simulink model "QuadrotorSimulink_no_memory"  (R2020a)
settings: Solver=FixedStepAuto  StartTime=0.0  StopTime=options.T_train  FixedStep=options.dt  RelTol=1e-6
undefined symbols (not defined in the file or in its folder): options, Quad
libraries: neural x67, simulink x1
(part 1 of 4)
settings Model: Creator=test  LastModifiedBy=kekatos
settings DataIOCC: LimitDataPoints=on  SaveFormat=Array  SignalLoggingSaveFormat=ModelDataLogs  ReturnWorkspaceOutputs=off
settings OptimizationCC: ExpressionDepthLimit=2147483647  LifeSpan=inf
settings DebuggingCC: UnderspecifiedInitializationDetection=Classic  MergeDetectMultiDrivingBlocksExec=none  SolverPrmCheckMsg=warning  FcnCallInpInsideContextMsg=warning  StateNameClashWarn=warning  SFUnexpectedBacktrackingDiag=warning  SFNoUnconditionalDefaultTransitionDiag=warning  SFExecutionAtInitializationDiag=none  ArithmeticOperatorsInVariantConditions=warning
settings HardwareCC: ProdBitPerPointer=32  ProdBitPerSizeT=32  ProdBitPerPtrDiffT=32  ProdLargestAtomicFloat=None  ProdIntDivRoundTo=Undefined  ProdEndianess=Unspecified  ProdWordSize=32  ProdHWDeviceType=32-bit Generic
settings ModelReferenceCC: PropagateSignalLabelsOutOfModel=off
settings SFSimCC: SimUseLocalCustomCode=off  CustomCodeUndefinedFunction=UseInterfaceOnly
settings RTWCC: RTWUseLocalCustomCode=off
settings CodeAppCC: StateflowObjectComments=on
settings GRTTargetCC: TargetLangStandard=C89/C90 (ANSI)  CombineOutputUpdateFcns=off  GRTInterface=on
settings ConfigComp: CovMetricSettings=dw  CovHtmlReporting=on  CovSaveCumulativeToWorkspaceVar=on  CovSaveSingleToWorkspaceVar=on

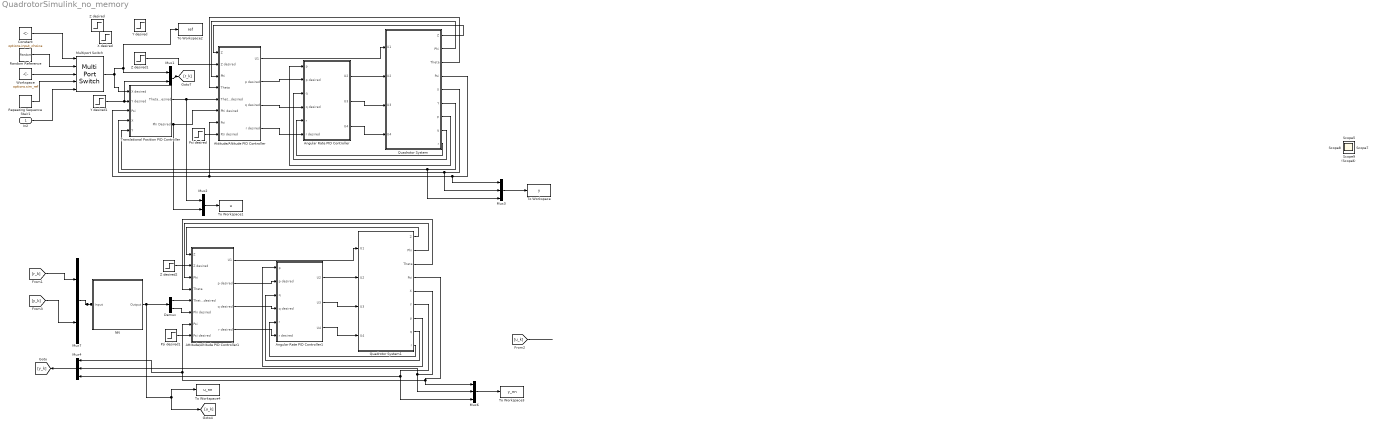
== system QuadrotorSimulink_no_memory ==
  In2 : Inport
  Angular Rate PID Controller : Subsystem
  Angular Rate PID Controller1 : Subsystem
  Attitude/Altitude PID Controller : Subsystem
  Attitude/Altitude PID Controller1 : Subsystem
  Constant : Constant  Value=options.input_choice
  Demux : Demux  Outputs=2
  Multiport Switch : MultiPortSwitch  Inputs=4
  Mux1 : Mux  Inputs=2
  Mux2 : Mux  Inputs=2
  Mux3 : Mux  Inputs=3
  Mux4 : Mux  Inputs=3
  Mux6 : Mux  Inputs=3
  Mux7 : Mux  Inputs=2
  NN : Subsystem
      mask help: Feed-Forward Neural Network
      mask Display: e = 0.06;c1 = [120 150 230]/255;c2 = ([120 150 230]+0)/383;c3 = ([120 150 230]+128)/383;patch([0 1 1 0],[0 0 1 1],c1);patch([0 1 1 1-e 1-e 0+e],[0 0 1 1-e 0+e 0+e],c2);patch([0 0 1 1-e 0+e 0+e],[0 1 1 1-e 1-e 0+e],c3);plot([0 1 1 0 0],[0 0 1 1 0]);fprintf('NNET');port_label('input',1,' Input');port_label('output',1,'Output ');
  Psi desired : Step  After=0  SampleTime=0
  Psi desired1 : Step  After=0  SampleTime=0
  Quadrotor System : Subsystem
  Quadrotor System1 : Subsystem
  Random Reference : UniformRandomNumber  Minimum=options.ref_min  Maximum=options.ref_max  Seed=randi(2^32,[1 ])  SampleTime=options.ref_Ts
  Repeating Sequence Stair1 : simulink/Sources/Repeating Sequence Stair  OutValues=options.sim_cov  tsamp=options.ref_Ts  OutMin=[]  OutMax=[]  OutDataTypeStr=double  OutputDataTypeScalingMode=double  OutDataType=fixdt(0,8)  ConRadixGroup=Best Precision: Vector-wise  OutScaling=2^-12
  To Workspace : ToWorkspace  VariableName=y  SaveFormat=Structure With Time  SampleTime=0.01
  To Workspace1 : ToWorkspace  VariableName=u  SaveFormat=Structure With Time  SampleTime=0.01
  To Workspace2 : ToWorkspace  VariableName=ref  SaveFormat=Structure With Time  SampleTime=0.01
  To Workspace3 : ToWorkspace  VariableName=y_nn  SaveFormat=Structure With Time  SampleTime=0.01
  To Workspace4 : ToWorkspace  VariableName=u_nn  SaveFormat=Structure With Time  SampleTime=0.01
  Translational Position PID Controller : Subsystem
  Workspace : Constant  Value=options.sim_ref
  X desired : Step  After=.25  SampleTime=0
  Y desired : Step  After=0  SampleTime=0
  Y desired1 : Step  Time=0  After=0.05  SampleTime=0
  Z desired : Step  After=.5  SampleTime=0
  Z desired1 : Step  Time=0  After=0.5  SampleTime=0
  Z desired2 : Step  Time=0  After=0.5  SampleTime=0
  Scope{,1..10} (11 alike) : Scope
  wires:
  Quadrotor System/2(Phi) -> Attitude/Altitude PID Controller/3(Phi)
  Quadrotor System/3(Theta) -> Attitude/Altitude PID Controller/4(Theta)
  Quadrotor System/4(Psi) -> Mux3/1, Translational Position PID Controller/3(Psi), Attitude/Altitude PID Controller/7(Psi)
  Quadrotor System/5(X) -> Mux3/2, Translational Position PID Controller/4(X)
  Quadrotor System/6(Y) -> Mux3/3, Translational Position PID Controller/5(Y)
  Quadrotor System/1(Z) -> Attitude/Altitude PID Controller/1(Z)
  Psi desired/1 -> Attitude/Altitude PID Controller/8(Psi desired)
  Attitude/Altitude PID Controller/1(U1) -> Quadrotor System/1(U1)
  Translational Position PID Controller/1(Theta Desired) -> Mux2/1, Attitude/Altitude PID Controller/5(Theta desired)
  Translational Position PID Controller/2(Phi Desired) -> Attitude/Altitude PID Controller/6(Phi desired), Mux2/2
  Attitude/Altitude PID Controller/2(p desired) -> Angular Rate PID Controller/2(p desired)
  Attitude/Altitude PID Controller/3(q desired) -> Angular Rate PID Controller/4(q desired)
  Attitude/Altitude PID Controller/4(r desired) -> Angular Rate PID Controller/6(r desired)
  Quadrotor System/9(r) -> Angular Rate PID Controller/5(r)
  Quadrotor System/8(q) -> Angular Rate PID Controller/3(q)
  Quadrotor System/7(p) -> Angular Rate PID Controller/1(p)
  Angular Rate PID Controller/3(U4) -> Quadrotor System/4(U4)
  Angular Rate PID Controller/2(U3) -> Quadrotor System/3(U3)
  Angular Rate PID Controller/1(U2) -> Quadrotor System/2(U2)
  Y desired1/1 -> Mux1/2, Translational Position PID Controller/2(Y desired)
  Z desired1/1 -> Attitude/Altitude PID Controller/2(Z desired)
  Mux2/1 -> To Workspace1/1
  Mux3/1 -> To Workspace/1
  In2/1 -> Multiport Switch/5
  Workspace/1 -> Multiport Switch/3
  Random Reference/1 -> Multiport Switch/2
  Repeating Sequence Stair1/1 -> Multiport Switch/4
  Constant/1 -> Multiport Switch/1
  Attitude/Altitude PID Controller1/2(p desired) -> Angular Rate PID Controller1/2(p desired)
  Attitude/Altitude PID Controller1/1(U1) -> Quadrotor System1/1(U1)
  Psi desired1/1 -> Attitude/Altitude PID Controller1/8(Psi desired)
  Quadrotor System1/9(r) -> Angular Rate PID Controller1/5(r)
  Quadrotor System1/6(Y) -> Mux4/3, Mux6/3
  Angular Rate PID Controller1/2(U3) -> Quadrotor System1/3(U3)
  Demux/1 -> Attitude/Altitude PID Controller1/5(Theta desired)
  Attitude/Altitude PID Controller1/3(q desired) -> Angular Rate PID Controller1/4(q desired)
  Quadrotor System1/7(p) -> Angular Rate PID Controller1/1(p)
  Quadrotor System1/2(Phi) -> Attitude/Altitude PID Controller1/3(Phi)
  Z desired2/1 -> Attitude/Altitude PID Controller1/2(Z desired)
  Quadrotor System1/4(Psi) -> Mux6/1, Mux4/1, Attitude/Altitude PID Controller1/7(Psi)
  Demux/2 -> Attitude/Altitude PID Controller1/6(Phi desired)
  Quadrotor System1/3(Theta) -> Attitude/Altitude PID Controller1/4(Theta)
  Angular Rate PID Controller1/1(U2) -> Quadrotor System1/2(U2)
  Quadrotor System1/5(X) -> Mux4/2, Mux6/2
  Angular Rate PID Controller1/3(U4) -> Quadrotor System1/4(U4)
  Quadrotor System1/1(Z) -> Attitude/Altitude PID Controller1/1(Z)
  Attitude/Altitude PID Controller1/4(r desired) -> Angular Rate PID Controller1/6(r desired)
  NN/1(Output) -> [u_k], To Workspace4/1, Demux/1
  Mux6/1 -> To Workspace3/1
  Quadrotor System1/8(q) -> Angular Rate PID Controller1/3(q)
  Mux7/1 -> NN/1(Input)
  Multiport Switch/1 -> Translational Position PID Controller/1(X desired), To Workspace2/1, Mux1/1
  Mux4/1 -> [y_k]
  [r_k] -> Mux7/1
  [u_k] -> ?
  Mux1/1 -> [r_k]
  [y_k] -> Mux7/2

== system QuadrotorSimulink_no_memory/Angular Rate PID Controller ==
  p : Inport
  p desired : Inport  Port=2
  q : Inport  Port=3
  q desired : Inport  Port=4
  r : Inport  Port=5
  r desired : Inport  Port=6
  p PID : Subsystem
  q PID : Subsystem
  r PID : Subsystem
  U2 : Outport  VectorParamsAs1DForOutWhenUnconnected=off
  U3 : Outport  Port=2  VectorParamsAs1DForOutWhenUnconnected=off
  U4 : Outport  Port=3  VectorParamsAs1DForOutWhenUnconnected=off
  wires:
  p PID/1(U2) -> U2/1
  q PID/1(U3) -> U3/1
  r PID/1(U4) -> U4/1
  p/1 -> p PID/1(p)
  p desired/1 -> p PID/2(p desired)
  q/1 -> q PID/1(q)
  q desired/1 -> q PID/2(q desired)
  r/1 -> r PID/1(r)
  r desired/1 -> r PID/2(r desired)

== system QuadrotorSimulink_no_memory/Angular Rate PID Controller1 ==
  p : Inport
  p desired : Inport  Port=2
  q : Inport  Port=3
  q desired : Inport  Port=4
  r : Inport  Port=5
  r desired : Inport  Port=6
  p PID : Subsystem
  q PID : Subsystem
  r PID : Subsystem
  U2 : Outport  VectorParamsAs1DForOutWhenUnconnected=off
  U3 : Outport  Port=2  VectorParamsAs1DForOutWhenUnconnected=off
  U4 : Outport  Port=3  VectorParamsAs1DForOutWhenUnconnected=off
  wires:
  p PID/1(U2) -> U2/1
  q PID/1(U3) -> U3/1
  r PID/1(U4) -> U4/1
  p/1 -> p PID/1(p)
  p desired/1 -> p PID/2(p desired)
  q/1 -> q PID/1(q)
  q desired/1 -> q PID/2(q desired)
  r/1 -> r PID/1(r)
  r desired/1 -> r PID/2(r desired)

== system QuadrotorSimulink_no_memory/Attitude//Altitude PID Controller ==
  Z : Inport
  Z desired : Inport  Port=2
  Phi : Inport  Port=3
  Theta : Inport  Port=4
  Theta desired : Inport  Port=5
  Phi desired : Inport  Port=6
  Psi : Inport  Port=7
  Psi desired : Inport  Port=8
  Phi PID : Subsystem
  Psi PID : Subsystem
  Theta PID : Subsystem
  Z PID : Subsystem
  U1 : Outport  VectorParamsAs1DForOutWhenUnconnected=off
  p desired : Outport  Port=2  VectorParamsAs1DForOutWhenUnconnected=off
  q desired : Outport  Port=3  VectorParamsAs1DForOutWhenUnconnected=off
  r desired : Outport  Port=4  VectorParamsAs1DForOutWhenUnconnected=off
  wires:
  Z PID/1(U1) -> U1/1
  Z desired/1 -> Z PID/2(Z desired)
  Z/1 -> Z PID/1(Z)
  Phi desired/1 -> Phi PID/2(Phi desired)
  Phi/1 -> Phi PID/1(Phi), Z PID/3(Phi)
  Psi desired/1 -> Psi PID/2(Psi desired)
  Psi/1 -> Psi PID/1(Psi)
  Theta desired/1 -> Theta PID/2(Theta desired)
  Theta/1 -> Theta PID/1(Theta), Z PID/4(Theta)
  Phi PID/1(p desired) -> p desired/1
  Psi PID/1(r desired) -> r desired/1
  Theta PID/1(q desired) -> q desired/1

== system QuadrotorSimulink_no_memory/Attitude//Altitude PID Controller1 ==
  Z : Inport
  Z desired : Inport  Port=2
  Phi : Inport  Port=3
  Theta : Inport  Port=4
  Theta desired : Inport  Port=5
  Phi desired : Inport  Port=6
  Psi : Inport  Port=7
  Psi desired : Inport  Port=8
  Phi PID : Subsystem
  Psi PID : Subsystem
  Theta PID : Subsystem
  Z PID : Subsystem
  U1 : Outport  VectorParamsAs1DForOutWhenUnconnected=off
  p desired : Outport  Port=2  VectorParamsAs1DForOutWhenUnconnected=off
  q desired : Outport  Port=3  VectorParamsAs1DForOutWhenUnconnected=off
  r desired : Outport  Port=4  VectorParamsAs1DForOutWhenUnconnected=off
  wires:
  Z PID/1(U1) -> U1/1
  Z desired/1 -> Z PID/2(Z desired)
  Z/1 -> Z PID/1(Z)
  Phi desired/1 -> Phi PID/2(Phi desired)
  Phi/1 -> Phi PID/1(Phi), Z PID/3(Phi)
  Psi desired/1 -> Psi PID/2(Psi desired)
  Psi/1 -> Psi PID/1(Psi)
  Theta desired/1 -> Theta PID/2(Theta desired)
  Theta/1 -> Theta PID/1(Theta), Z PID/4(Theta)
  Phi PID/1(p desired) -> p desired/1
  Psi PID/1(r desired) -> r desired/1
  Theta PID/1(q desired) -> q desired/1

== system QuadrotorSimulink_no_memory/NN ==
  Input : Inport  PortDimensions=5
      mask Display: e = 0.06;c1 = [120 230 180]/255;c2 = ([120 230 180]+0)/(256+128);c3 = ([120 230 180]+128)/(256+128);patch([0 1 1 0],[0 0 1 1],c1);patch([0 1 1 1-e 1-e 0+e],[0 0 1 1-e 0+e 0+e],c2);patch([0 0 1 1-e 0+e 0+e],[0 1 1 1-e 1-e 0+e],c3);plot([0 1 1 0 0],[0 0 1 1 0]);
  Layer 1 : Subsystem
      mask Display: e = 0.06;c1 = [120 150 230]/255;c2 = ([120 150 230]+0)/383;c3 = ([120 150 230]+128)/383;patch([0 1 1 0],[0 0 1 1],c1);patch([0 1 1 1-e 1-e 0+e],[0 0 1 1-e 0+e 0+e],c2);patch([0 0 1 1-e 0+e 0+e],[0 1 1 1-e 1-e 0+e],c3);plot([0 1 1 0 0],[0 0 1 1 0]);
  Layer 2 : Subsystem
      mask Display: e = 0.06;c1 = [120 150 230]/255;c2 = ([120 150 230]+0)/383;c3 = ([120 150 230]+128)/383;patch([0 1 1 0],[0 0 1 1],c1);patch([0 1 1 1-e 1-e 0+e],[0 0 1 1-e 0+e 0+e],c2);patch([0 0 1 1-e 0+e 0+e],[0 1 1 1-e 1-e 0+e],c3);plot([0 1 1 0 0],[0 0 1 1 0]);
  Layer 3 : Subsystem
      mask Display: e = 0.06;c1 = [120 150 230]/255;c2 = ([120 150 230]+0)/383;c3 = ([120 150 230]+128)/383;patch([0 1 1 0],[0 0 1 1],c1);patch([0 1 1 1-e 1-e 0+e],[0 0 1 1-e 0+e 0+e],c2);patch([0 0 1 1-e 0+e 0+e],[0 1 1 1-e 1-e 0+e],c3);plot([0 1 1 0 0],[0 0 1 1 0]);
  Process Input 1 : Subsystem
      mask Display: e = 0.06;c1 = [120 150 230]/255;c2 = ([120 150 230]+0)/383;c3 = ([120 150 230]+128)/383;patch([0 1 1 0],[0 0 1 1],c1);patch([0 1 1 1-e 1-e 0+e],[0 0 1 1-e 0+e 0+e],c2);patch([0 0 1 1-e 0+e 0+e],[0 1 1 1-e 1-e 0+e],c3);plot([0 1 1 0 0],[0 0 1 1 0]);
  Process Output 1 : Subsystem
      mask Display: e = 0.06;c1 = [120 150 230]/255;c2 = ([120 150 230]+0)/383;c3 = ([120 150 230]+128)/383;patch([0 1 1 0],[0 0 1 1],c1);patch([0 1 1 1-e 1-e 0+e],[0 0 1 1-e 0+e 0+e],c2);patch([0 0 1 1-e 0+e 0+e],[0 1 1 1-e 1-e 0+e],c3);plot([0 1 1 0 0],[0 0 1 1 0]);
  Output : Outport  InitialOutput=[0;0]
      mask Display: e = 0.06;c1 = [120 230 180]/255;c2 = ([120 230 180]+0)/(256+128);c3 = ([120 230 180]+128)/(256+128);patch([0 1 1 0],[0 0 1 1],c1);patch([0 1 1 1-e 1-e 0+e],[0 0 1 1-e 0+e 0+e],c2);patch([0 0 1 1-e 0+e 0+e],[0 1 1 1-e 1-e 0+e],c3);plot([0 1 1 0 0],[0 0 1 1 0]);
  wires:
  Input/1 -> Process Input 1/1(x)
  Process Output 1/1(y) -> Output/1
  Process Input 1/1(p) -> Layer 1/1("p{1}")
  Layer 1/1("a{1}") -> [feedback1]
  [feedback1] -> Layer 2/1("a{1} ")
  Layer 2/1("a{2}") -> [feedback2]
  [feedback2] -> Layer 3/1("a{2} ")
  Layer 3/1("a{3}") -> Process Output 1/1(a)

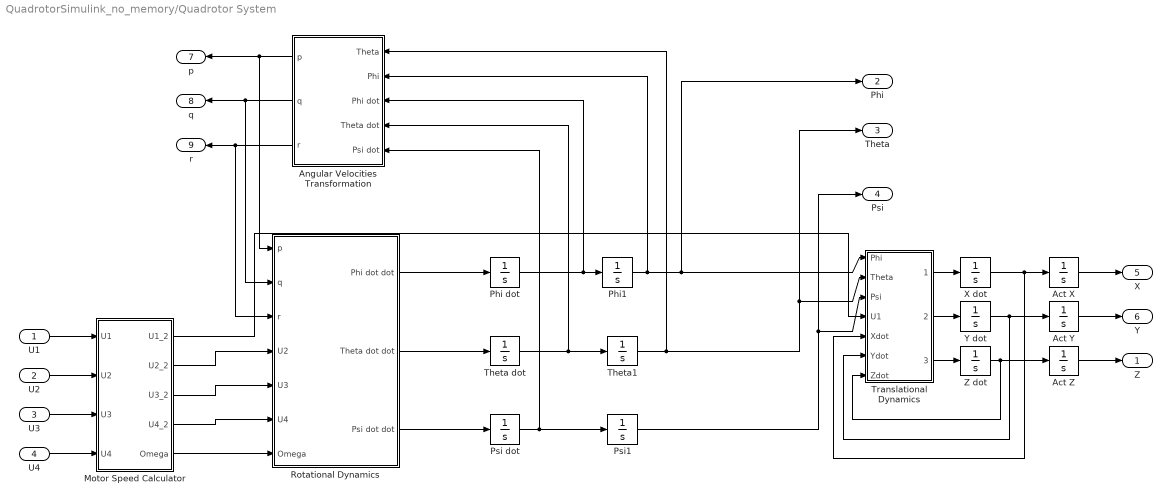
== system QuadrotorSimulink_no_memory/Quadrotor System ==
  U1 : Inport
  U2 : Inport  Port=2
  U3 : Inport  Port=3
  U4 : Inport  Port=4
  Act X : Integrator
  Act Y : Integrator
  Act Z : Integrator
  Angular Velocities Transformation : Subsystem
  Motor Speed Calculator : Subsystem
  Phi dot : Integrator
  Phi1 : Integrator  ZeroCross=off
  Psi dot : Integrator  ZeroCross=off
  Psi1 : Integrator  ZeroCross=off
  Rotational Dynamics : Subsystem
  Theta dot : Integrator  ZeroCross=off
  Theta1 : Integrator  ZeroCross=off
  Translational Dynamics : Subsystem
  X dot : Integrator
  Y dot : Integrator
  Z dot : Integrator
  Z : Outport  VectorParamsAs1DForOutWhenUnconnected=off
  Phi : Outport  Port=2  VectorParamsAs1DForOutWhenUnconnected=off
  Theta : Outport  Port=3  VectorParamsAs1DForOutWhenUnconnected=off
  Psi : Outport  Port=4  VectorParamsAs1DForOutWhenUnconnected=off
  X : Outport  Port=5  VectorParamsAs1DForOutWhenUnconnected=off
  Y : Outport  Port=6  VectorParamsAs1DForOutWhenUnconnected=off
  p : Outport  Port=7  VectorParamsAs1DForOutWhenUnconnected=off
  q : Outport  Port=8  VectorParamsAs1DForOutWhenUnconnected=off
  r : Outport  Port=9  VectorParamsAs1DForOutWhenUnconnected=off
  wires:
  Rotational Dynamics/2(Theta dot dot) -> Theta dot/1
  Motor Speed Calculator/5(Omega) -> Rotational Dynamics/7(Omega)
  Phi1/1 -> Translational Dynamics/1(Phi), Phi/1, Angular Velocities Transformation/2(Phi)
  Theta1/1 -> Translational Dynamics/2(Theta), Theta/1, Angular Velocities Transformation/1(Theta)
  Psi1/1 -> Translational Dynamics/3(Psi), Psi/1
  Translational Dynamics/1(x dotdot) -> X dot/1
  X dot/1 -> Act X/1, Translational Dynamics/5(Xdot)
  Y dot/1 -> Act Y/1, Translational Dynamics/6(Ydot)
  Translational Dynamics/2(y dotdot) -> Y dot/1
  Z dot/1 -> Translational Dynamics/7(Zdot), Act Z/1
  Translational Dynamics/3(z dotdot) -> Z dot/1
  Act X/1 -> X/1
  Act Y/1 -> Y/1
  Act Z/1 -> Z/1
  Psi dot/1 -> Psi1/1, Angular Velocities Transformation/5(Psi dot)
  Theta dot/1 -> Theta1/1, Angular Velocities Transformation/4(Theta dot)
  Phi dot/1 -> Phi1/1, Angular Velocities Transformation/3(Phi dot)
  Rotational Dynamics/3(Psi dot dot) -> Psi dot/1
  Rotational Dynamics/1(Phi dot dot) -> Phi dot/1
  U4/1 -> Motor Speed Calculator/4(U4)
  U2/1 -> Motor Speed Calculator/2(U2)
  U3/1 -> Motor Speed Calculator/3(U3)
  Motor Speed Calculator/2(U2_2) -> Rotational Dynamics/4(U2)
  Motor Speed Calculator/3(U3_2) -> Rotational Dynamics/5(U3)
  Motor Speed Calculator/1(U1_2) -> Translational Dynamics/4(U1)
  Motor Speed Calculator/4(U4_2) -> Rotational Dynamics/6(U4)
  Angular Velocities Transformation/1(p) -> Rotational Dynamics/1(p), p/1
  Angular Velocities Transformation/2(q) -> Rotational Dynamics/2(q), q/1
  Angular Velocities Transformation/3(r) -> Rotational Dynamics/3(r), r/1
  U1/1 -> Motor Speed Calculator/1(U1)

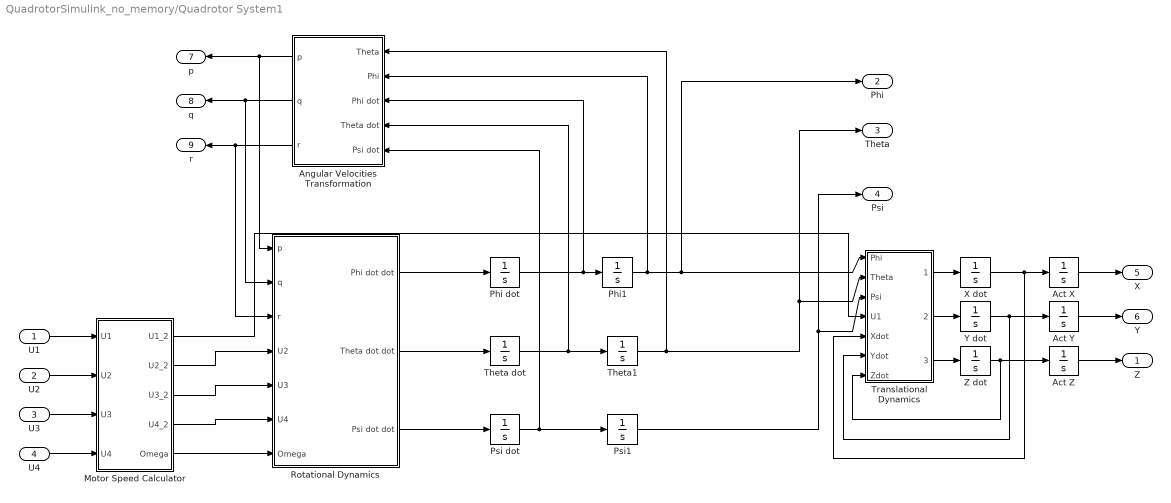
== system QuadrotorSimulink_no_memory/Quadrotor System1 ==
  U1 : Inport
  U2 : Inport  Port=2
  U3 : Inport  Port=3
  U4 : Inport  Port=4
  Act X : Integrator
  Act Y : Integrator
  Act Z : Integrator
  Angular Velocities Transformation : Subsystem
  Motor Speed Calculator : Subsystem
  Phi dot : Integrator
  Phi1 : Integrator  ZeroCross=off
  Psi dot : Integrator  ZeroCross=off
  Psi1 : Integrator  ZeroCross=off
  Rotational Dynamics : Subsystem
  Theta dot : Integrator  ZeroCross=off
  Theta1 : Integrator  ZeroCross=off
  Translational Dynamics : Subsystem
  X dot : Integrator
  Y dot : Integrator
  Z dot : Integrator
  Z : Outport  VectorParamsAs1DForOutWhenUnconnected=off
  Phi : Outport  Port=2  VectorParamsAs1DForOutWhenUnconnected=off
  Theta : Outport  Port=3  VectorParamsAs1DForOutWhenUnconnected=off
  Psi : Outport  Port=4  VectorParamsAs1DForOutWhenUnconnected=off
  X : Outport  Port=5  VectorParamsAs1DForOutWhenUnconnected=off
  Y : Outport  Port=6  VectorParamsAs1DForOutWhenUnconnected=off
  p : Outport  Port=7  VectorParamsAs1DForOutWhenUnconnected=off
  q : Outport  Port=8  VectorParamsAs1DForOutWhenUnconnected=off
  r : Outport  Port=9  VectorParamsAs1DForOutWhenUnconnected=off
  wires:
  Rotational Dynamics/2(Theta dot dot) -> Theta dot/1
  Motor Speed Calculator/5(Omega) -> Rotational Dynamics/7(Omega)
  Phi1/1 -> Translational Dynamics/1(Phi), Phi/1, Angular Velocities Transformation/2(Phi)
  Theta1/1 -> Translational Dynamics/2(Theta), Theta/1, Angular Velocities Transformation/1(Theta)
  Psi1/1 -> Translational Dynamics/3(Psi), Psi/1
  Translational Dynamics/1(x dotdot) -> X dot/1
  X dot/1 -> Act X/1, Translational Dynamics/5(Xdot)
  Y dot/1 -> Act Y/1, Translational Dynamics/6(Ydot)
  Translational Dynamics/2(y dotdot) -> Y dot/1
  Z dot/1 -> Translational Dynamics/7(Zdot), Act Z/1
  Translational Dynamics/3(z dotdot) -> Z dot/1
  Act X/1 -> X/1
  Act Y/1 -> Y/1
  Act Z/1 -> Z/1
  Psi dot/1 -> Psi1/1, Angular Velocities Transformation/5(Psi dot)
  Theta dot/1 -> Theta1/1, Angular Velocities Transformation/4(Theta dot)
  Phi dot/1 -> Phi1/1, Angular Velocities Transformation/3(Phi dot)
  Rotational Dynamics/3(Psi dot dot) -> Psi dot/1
  Rotational Dynamics/1(Phi dot dot) -> Phi dot/1
  U4/1 -> Motor Speed Calculator/4(U4)
  U2/1 -> Motor Speed Calculator/2(U2)
  U3/1 -> Motor Speed Calculator/3(U3)
  Motor Speed Calculator/2(U2_2) -> Rotational Dynamics/4(U2)
  Motor Speed Calculator/3(U3_2) -> Rotational Dynamics/5(U3)
  Motor Speed Calculator/1(U1_2) -> Translational Dynamics/4(U1)
  Motor Speed Calculator/4(U4_2) -> Rotational Dynamics/6(U4)
  Angular Velocities Transformation/1(p) -> Rotational Dynamics/1(p), p/1
  Angular Velocities Transformation/2(q) -> Rotational Dynamics/2(q), q/1
  Angular Velocities Transformation/3(r) -> Rotational Dynamics/3(r), r/1
  U1/1 -> Motor Speed Calculator/1(U1)

== system QuadrotorSimulink_no_memory/Translational Position PID Controller ==
  X desired : Inport
  Y desired : Inport  Port=2
  Psi : Inport  Port=3
  X : Inport  Port=4
  Y : Inport  Port=5
  Desired Position GF to BF : Subsystem
  Position GF to BF : Subsystem
  X PID : Subsystem
  Y PID : Subsystem
  Theta Desired : Outport  VectorParamsAs1DForOutWhenUnconnected=off
  Phi Desired : Outport  Port=2  VectorParamsAs1DForOutWhenUnconnected=off
  wires:
  X PID/1(Theta Desired) -> Theta Desired/1
  Y PID/1(Phi Desired) -> Phi Desired/1
  X desired/1 -> Desired Position GF to BF/1(X GF)
  Y desired/1 -> Desired Position GF to BF/2(Y GF)
  Desired Position GF to BF/1("X Bf ") -> X PID/1(X desired)
  Desired Position GF to BF/2(Y Bf) -> Y PID/1(Y desired)
  X/1 -> Position GF to BF/1(X GF)
  Y/1 -> Position GF to BF/2(Y GF)
  Position GF to BF/1("X Bf ") -> X PID/2(X)
  Position GF to BF/2(Y Bf) -> Y PID/2(Y)
  Psi/1 -> Desired Position GF to BF/3(Psi), Position GF to BF/3(Psi)

== system QuadrotorSimulink_no_memory/Angular Rate PID Controller/p PID ==
  p : Inport
  p desired : Inport  Port=2
  Derivative : Derivative
  Integrator : Integrator
  Kd : Gain  Gain=Quad.p_KD
  Ki : Gain  Gain=Quad.p_KI
  Kp : Gain  Gain=Quad.p_KP
  Psi Error : Sum  Inputs=+-
  Saturation1 : Saturate  UpperLimit=Quad.U2_max  LowerLimit=Quad.U2_min
  Sum : Sum  Inputs=+++
  U2 : Outport  VectorParamsAs1DForOutWhenUnconnected=off
  wires:
  p/1 -> Psi Error/2, Derivative/1
  p desired/1 -> Psi Error/1
  Derivative/1 -> Kd/1
  Kp/1 -> Sum/1
  Sum/1 -> U2/1
  Psi Error/1 -> Integrator/1, Kp/1
  Integrator/1 -> Ki/1
  Kd/1 -> Sum/3
  Ki/1 -> Saturation1/1
  Saturation1/1 -> Sum/2

== system QuadrotorSimulink_no_memory/Angular Rate PID Controller/q PID ==
  q : Inport
  q desired : Inport  Port=2
  Derivative : Derivative
  Integrator : Integrator
  Kd : Gain  Gain=Quad.q_KD
  Ki : Gain  Gain=Quad.q_KI
  Kp : Gain  Gain=Quad.q_KP
  Saturation1 : Saturate  UpperLimit=Quad.U3_max  LowerLimit=Quad.U3_min
  Scope : Scope
  Sum : Sum  Inputs=+++
  q Error : Sum  Inputs=+-
  U3 : Outport  VectorParamsAs1DForOutWhenUnconnected=off
  wires:
  q/1 -> q Error/2, Derivative/1
  q desired/1 -> q Error/1
  Derivative/1 -> Kd/1
  Kp/1 -> Sum/1
  Sum/1 -> U3/1
  q Error/1 -> Integrator/1, Kp/1, Scope/1
  Integrator/1 -> Ki/1
  Kd/1 -> Sum/3
  Ki/1 -> Saturation1/1
  Saturation1/1 -> Sum/2

== system QuadrotorSimulink_no_memory/Angular Rate PID Controller/r PID ==
  r : Inport
  r desired : Inport  Port=2
  Derivative : Derivative
  Integrator : Integrator
  Kd : Gain  Gain=Quad.r_KD
  Ki : Gain  Gain=Quad.r_KI
  Kp : Gain  Gain=Quad.r_KP
  Psi Error : Sum  Inputs=+-
  Sum : Sum  Inputs=+++
  U4 : Outport  VectorParamsAs1DForOutWhenUnconnected=off
  wires:
  r/1 -> Psi Error/2, Derivative/1
  r desired/1 -> Psi Error/1
  Derivative/1 -> Kd/1
  Kp/1 -> Sum/1
  Sum/1 -> U4/1
  Psi Error/1 -> Integrator/1, Kp/1
  Integrator/1 -> Ki/1
  Kd/1 -> Sum/3

== system QuadrotorSimulink_no_memory/Angular Rate PID Controller1/p PID ==
  p : Inport
  p desired : Inport  Port=2
  Derivative : Derivative
  Integrator : Integrator
  Kd : Gain  Gain=Quad.p_KD
  Ki : Gain  Gain=Quad.p_KI
  Kp : Gain  Gain=Quad.p_KP
  Psi Error : Sum  Inputs=+-
  Saturation1 : Saturate  UpperLimit=Quad.U2_max  LowerLimit=Quad.U2_min
  Sum : Sum  Inputs=+++
  U2 : Outport  VectorParamsAs1DForOutWhenUnconnected=off
  wires:
  p/1 -> Psi Error/2, Derivative/1
  p desired/1 -> Psi Error/1
  Derivative/1 -> Kd/1
  Kp/1 -> Sum/1
  Sum/1 -> U2/1
  Psi Error/1 -> Integrator/1, Kp/1
  Integrator/1 -> Ki/1
  Kd/1 -> Sum/3
  Ki/1 -> Saturation1/1
  Saturation1/1 -> Sum/2

== system QuadrotorSimulink_no_memory/Angular Rate PID Controller1/q PID ==
  q : Inport
  q desired : Inport  Port=2
  Derivative : Derivative
  Integrator : Integrator
  Kd : Gain  Gain=Quad.q_KD
  Ki : Gain  Gain=Quad.q_KI
  Kp : Gain  Gain=Quad.q_KP
  Saturation1 : Saturate  UpperLimit=Quad.U3_max  LowerLimit=Quad.U3_min
  Scope : Scope
  Sum : Sum  Inputs=+++
  q Error : Sum  Inputs=+-
  U3 : Outport  VectorParamsAs1DForOutWhenUnconnected=off
  wires:
  q/1 -> q Error/2, Derivative/1
  q desired/1 -> q Error/1
  Derivative/1 -> Kd/1
  Kp/1 -> Sum/1
  Sum/1 -> U3/1
  q Error/1 -> Integrator/1, Kp/1, Scope/1
  Integrator/1 -> Ki/1
  Kd/1 -> Sum/3
  Ki/1 -> Saturation1/1
  Saturation1/1 -> Sum/2

== system QuadrotorSimulink_no_memory/Angular Rate PID Controller1/r PID ==
  r : Inport
  r desired : Inport  Port=2
  Derivative : Derivative
  Integrator : Integrator
  Kd : Gain  Gain=Quad.r_KD
  Ki : Gain  Gain=Quad.r_KI
  Kp : Gain  Gain=Quad.r_KP
  Psi Error : Sum  Inputs=+-
  Sum : Sum  Inputs=+++
  U4 : Outport  VectorParamsAs1DForOutWhenUnconnected=off
  wires:
  r/1 -> Psi Error/2, Derivative/1
  r desired/1 -> Psi Error/1
  Derivative/1 -> Kd/1
  Kp/1 -> Sum/1
  Sum/1 -> U4/1
  Psi Error/1 -> Integrator/1, Kp/1
  Integrator/1 -> Ki/1
  Kd/1 -> Sum/3

== system QuadrotorSimulink_no_memory/Attitude//Altitude PID Controller/Phi PID ==
  Phi : Inport
  Phi desired : Inport  Port=2
  Derivative : Derivative
  Integrator : Integrator
  Kd : Gain  Gain=Quad.phi_KD
  Ki : Gain  Gain=Quad.phi_KI
  Kp : Gain  Gain=Quad.phi_KP
  Psi Error : Sum  Inputs=+-
  Sum : Sum  Inputs=+++
  p desired : Outport  VectorParamsAs1DForOutWhenUnconnected=off
  wires:
  Phi/1 -> Psi Error/2, Derivative/1
  Phi desired/1 -> Psi Error/1
  Derivative/1 -> Kd/1
  Kp/1 -> Sum/1
  Sum/1 -> p desired/1
  Psi Error/1 -> Integrator/1, Kp/1
  Integrator/1 -> Ki/1
  Kd/1 -> Sum/3
  Ki/1 -> Sum/2

== system QuadrotorSimulink_no_memory/Attitude//Altitude PID Controller/Psi PID ==
  Psi : Inport
  Psi desired : Inport  Port=2
  Derivative : Derivative
  Integrator : Integrator
  Kd : Gain  Gain=Quad.psi_KD
  Ki : Gain  Gain=Quad.psi_KI
  Kp : Gain  Gain=Quad.psi_KP
  Psi Error : Sum  Inputs=+-
  Sum : Sum  Inputs=+++
  r desired : Outport  VectorParamsAs1DForOutWhenUnconnected=off
  wires:
  Psi/1 -> Psi Error/2, Derivative/1
  Psi desired/1 -> Psi Error/1
  Derivative/1 -> Kd/1
  Kp/1 -> Sum/1
  Sum/1 -> r desired/1
  Psi Error/1 -> Integrator/1, Kp/1
  Integrator/1 -> Ki/1
  Kd/1 -> Sum/3
  Ki/1 -> Sum/2

== system QuadrotorSimulink_no_memory/Attitude//Altitude PID Controller/Theta PID ==
  Theta : Inport
  Theta desired : Inport  Port=2
  Derivative : Derivative
  Integrator : Integrator
  Kd : Gain  Gain=Quad.theta_KD
  Ki : Gain  Gain=Quad.theta_KI
  Kp : Gain  Gain=Quad.theta_KP
  Scope : Scope
  Sum : Sum  Inputs=+++
  Theta Error : Sum  Inputs=+-
  q desired : Outport  VectorParamsAs1DForOutWhenUnconnected=off
  wires:
  Theta/1 -> Theta Error/2, Derivative/1
  Theta desired/1 -> Theta Error/1
  Derivative/1 -> Kd/1
  Kp/1 -> Sum/1
  Sum/1 -> q desired/1
  Theta Error/1 -> Integrator/1, Kp/1, Scope/1
  Integrator/1 -> Ki/1
  Kd/1 -> Sum/3
  Ki/1 -> Sum/2

== system QuadrotorSimulink_no_memory/Attitude//Altitude PID Controller/Z PID ==
  Z : Inport
  Z desired : Inport  Port=2
  Phi : Inport  Port=3
  Theta : Inport  Port=4
  Derivative : Derivative
  Divide : Product  Inputs=*/
  Integrator : Integrator
  Kd : Gain  Gain=Quad.Z_KD
  Ki : Gain  Gain=Quad.Z_KI
  Kp : Gain  Gain=Quad.Z_KP
  Product : Product  RndMeth=Zero
  Sum : Sum  Inputs=---+
  cos Phi : Trigonometry  Operator=cos
  cos Theta : Trigonometry  Operator=cos
  ez : Sum  Inputs=+-
  mg : Constant  Value=Quad.m*Quad.g
  U1 : Outport  VectorParamsAs1DForOutWhenUnconnected=off
  wires:
  Z desired/1 -> ez/1
  cos Phi/1 -> Product/1
  cos Theta/1 -> Product/2
  Product/1 -> Divide/2
  Phi/1 -> cos Phi/1
  Theta/1 -> cos Theta/1
  Z/1 -> ez/2, Derivative/1
  Derivative/1 -> Kd/1
  Kp/1 -> Sum/1
  Integrator/1 -> Ki/1
  ez/1 -> Integrator/1, Kp/1
  Sum/1 -> Divide/1
  Divide/1 -> U1/1
  mg/1 -> Sum/4
  Kd/1 -> Sum/3
  Ki/1 -> Sum/2

== system QuadrotorSimulink_no_memory/Attitude//Altitude PID Controller1/Phi PID ==
  Phi : Inport
  Phi desired : Inport  Port=2
  Derivative : Derivative
  Integrator : Integrator
  Kd : Gain  Gain=Quad.phi_KD
  Ki : Gain  Gain=Quad.phi_KI
  Kp : Gain  Gain=Quad.phi_KP
  Psi Error : Sum  Inputs=+-
  Sum : Sum  Inputs=+++
  p desired : Outport  VectorParamsAs1DForOutWhenUnconnected=off
  wires:
  Phi/1 -> Psi Error/2, Derivative/1
  Phi desired/1 -> Psi Error/1
  Derivative/1 -> Kd/1
  Kp/1 -> Sum/1
  Sum/1 -> p desired/1
  Psi Error/1 -> Integrator/1, Kp/1
  Integrator/1 -> Ki/1
  Kd/1 -> Sum/3
  Ki/1 -> Sum/2

== system QuadrotorSimulink_no_memory/Attitude//Altitude PID Controller1/Psi PID ==
  Psi : Inport
  Psi desired : Inport  Port=2
  Derivative : Derivative
  Integrator : Integrator
  Kd : Gain  Gain=Quad.psi_KD
  Ki : Gain  Gain=Quad.psi_KI
  Kp : Gain  Gain=Quad.psi_KP
  Psi Error : Sum  Inputs=+-
  Sum : Sum  Inputs=+++
  r desired : Outport  VectorParamsAs1DForOutWhenUnconnected=off
  wires:
  Psi/1 -> Psi Error/2, Derivative/1
  Psi desired/1 -> Psi Error/1
  Derivative/1 -> Kd/1
  Kp/1 -> Sum/1
  Sum/1 -> r desired/1
  Psi Error/1 -> Integrator/1, Kp/1
  Integrator/1 -> Ki/1
  Kd/1 -> Sum/3
  Ki/1 -> Sum/2

== system QuadrotorSimulink_no_memory/Attitude//Altitude PID Controller1/Theta PID ==
  Theta : Inport
  Theta desired : Inport  Port=2
  Derivative : Derivative
  Integrator : Integrator
  Kd : Gain  Gain=Quad.theta_KD
  Ki : Gain  Gain=Quad.theta_KI
  Kp : Gain  Gain=Quad.theta_KP
  Scope : Scope
  Sum : Sum  Inputs=+++
  Theta Error : Sum  Inputs=+-
  q desired : Outport  VectorParamsAs1DForOutWhenUnconnected=off
  wires:
  Theta/1 -> Theta Error/2, Derivative/1
  Theta desired/1 -> Theta Error/1
  Derivative/1 -> Kd/1
  Kp/1 -> Sum/1
  Sum/1 -> q desired/1
  Theta Error/1 -> Integrator/1, Kp/1, Scope/1
  Integrator/1 -> Ki/1
  Kd/1 -> Sum/3
  Ki/1 -> Sum/2

== system QuadrotorSimulink_no_memory/Attitude//Altitude PID Controller1/Z PID ==
  Z : Inport
  Z desired : Inport  Port=2
  Phi : Inport  Port=3
  Theta : Inport  Port=4
  Derivative : Derivative
  Divide : Product  Inputs=*/
  Integrator : Integrator
  Kd : Gain  Gain=Quad.Z_KD
  Ki : Gain  Gain=Quad.Z_KI
  Kp : Gain  Gain=Quad.Z_KP
  Product : Product  RndMeth=Zero
  Sum : Sum  Inputs=---+
  cos Phi : Trigonometry  Operator=cos
  cos Theta : Trigonometry  Operator=cos
  ez : Sum  Inputs=+-
  mg : Constant  Value=Quad.m*Quad.g
  U1 : Outport  VectorParamsAs1DForOutWhenUnconnected=off
  wires:
  Z desired/1 -> ez/1
  cos Phi/1 -> Product/1
  cos Theta/1 -> Product/2
  Product/1 -> Divide/2
  Phi/1 -> cos Phi/1
  Theta/1 -> cos Theta/1
  Z/1 -> ez/2, Derivative/1
  Derivative/1 -> Kd/1
  Kp/1 -> Sum/1
  Integrator/1 -> Ki/1
  ez/1 -> Integrator/1, Kp/1
  Sum/1 -> Divide/1
  Divide/1 -> U1/1
  mg/1 -> Sum/4
  Kd/1 -> Sum/3
  Ki/1 -> Sum/2

== system QuadrotorSimulink_no_memory/NN/Layer 1 ==
  "p{1}" : Inport  PortDimensions=5
      mask Display: e = 0.06;c1 = [120 230 180]/255;c2 = ([120 230 180]+0)/(256+128);c3 = ([120 230 180]+128)/(256+128);patch([0 1 1 0],[0 0 1 1],c1);patch([0 1 1 1-e 1-e 0+e],[0 0 1 1-e 0+e 0+e],c2);patch([0 0 1 1-e 0+e 0+e],[0 1 1 1-e 1-e 0+e],c3);plot([0 1 1 0 0],[0 0 1 1 0]);
  Delays 1 : Subsystem
      mask Display: e = 0.06;c1 = [120 150 230]/255;c2 = ([120 150 230]+0)/383;c3 = ([120 150 230]+128)/383;patch([0 1 1 0],[0 0 1 1],c1);patch([0 1 1 1-e 1-e 0+e],[0 0 1 1-e 0+e 0+e],c2);patch([0 0 1 1-e 0+e 0+e],[0 1 1 1-e 1-e 0+e],c3);plot([0 1 1 0 0],[0 0 1 1 0]);disp('0');
  "IW{1,1}" : Subsystem
      mask Display: e = 0.06;c1 = [120 150 230]/255;c2 = ([120 150 230]+0)/383;c3 = ([120 150 230]+128)/383;patch([0 1 1 0],[0 0 1 1],c1);patch([0 1 1 1-e 1-e 0+e],[0 0 1 1-e 0+e 0+e],c2);patch([0 0 1 1-e 0+e 0+e],[0 1 1 1-e 1-e 0+e],c3);plot([0 1 1 0 0],[0 0 1 1 0]);disp('W');
  "b{1}" : Constant  Value=[-2.974020024097197012480364719522185623645782470703125;-2.408557229058040594082967800204642117023468017578125;1.9826251064210558272549178582266904413700103759765625;-2.253797420224197711746683125966228544712066650390625;-1.69301762578659964475491506163962185382843017578125;-2.01714731969397487176820504828356206417083740234375;1.5765749225424661172922924379236064851284027099609375;1.534624120855574869182191832805983722209930419921875;-1.0733067293699780631044404799467884004116058349609375;-1.25322723113531520056085355463437736034393310546875;0.82773685832683929763931018896983005106449127197265625;-0.4930380791671165052747483059647493064403533935546875;0.8892879956922377093775367029593326151371002197265625;-0.441726324120570723597012374739279039204120635986328125;-0.0311575986485864327157901954024055157788097858428955078125;0.08117969601236231513841090645655640400946140289306640625;0.0176137082644802385467119876238939468748867511749267578125;-0.4254050013595731538629252099781297147274017333984375;0.9465923230761379425501900186645798385143280029296875;-1.82629678779627990792278069420717656612396240234375;0.61800463200910471517346422842820174992084503173828125;1.483819260077808621645090170204639434814453125;1.259240993584011647499210084788501262664794921875;-1.7645309222460550113709132347139529883861541748046875;1.58466766614025811321653236518613994121551513671875;1.865809745884555059802778487210161983966827392578125;-2.008758277619576038119930672110058367252349853515625;-2.66868914669106604975468144402839243412017822265625;-2.65921974015566053850534444791264832019805908203125;2.8916743981935422169726734864525496959686279296875]
      mask Display: e = 0.06;c1 = [120 150 230]/255;c2 = ([120 150 230]+0)/383;c3 = ([120 150 230]+128)/383;patch([0 1 1 0],[0 0 1 1],c1);patch([0 1 1 1-e 1-e 0+e],[0 0 1 1-e 0+e 0+e],c2);patch([0 0 1 1-e 0+e 0+e],[0 1 1 1-e 1-e 0+e],c3);plot([0 1 1 0 0],[0 0 1 1 0]);disp('b');
  netsum : Sum  Inputs=2  InputSameDT=on  SaturateOnIntegerOverflow=on  OutDataTypeStr=Inherit: Same as first input
      mask Display: e = 0.06;c1 = [120 150 230]/255;c2 = ([120 150 230]+0)/383;c3 = ([120 150 230]+128)/383;patch([0 1 1 0],[0 0 1 1],c1);patch([0 1 1 1-e 1-e 0+e],[0 0 1 1-e 0+e 0+e],c2);patch([0 0 1 1-e 0+e 0+e],[0 1 1 1-e 1-e 0+e],c3);plot([0 1 1 0 0],[0 0 1 1 0]);disp('+');
  tansig : neural/Transfer Functions/tansig
  "a{1}" : Outport  InitialOutput=[0;0;0;0;0;0;0;0;0;0;0;0;0;0;0;0;0;0;0;0;0;0;0;0;0;0;0;0;0;0]
      mask Display: e = 0.06;c1 = [120 230 180]/255;c2 = ([120 230 180]+0)/(256+128);c3 = ([120 230 180]+128)/(256+128);patch([0 1 1 0],[0 0 1 1],c1);patch([0 1 1 1-e 1-e 0+e],[0 0 1 1-e 0+e 0+e],c2);patch([0 0 1 1-e 0+e 0+e],[0 1 1 1-e 1-e 0+e],c3);plot([0 1 1 0 0],[0 0 1 1 0]);
  wires:
  "p{1}"/1 -> Delays 1/1("p{1}")
  Delays 1/1("pd{1,1}") -> "IW{1,1}"/1("pd{1,1}")
  "IW{1,1}"/1("iz{1,1}") -> netsum/1
  "b{1}"/1 -> netsum/2
  netsum/1 -> tansig/1
  tansig/1 -> "a{1}"/1

== system QuadrotorSimulink_no_memory/NN/Layer 2 ==
  "a{1} " : Inport  PortDimensions=30
      mask Display: e = 0.06;c1 = [120 230 180]/255;c2 = ([120 230 180]+0)/(256+128);c3 = ([120 230 180]+128)/(256+128);patch([0 1 1 0],[0 0 1 1],c1);patch([0 1 1 1-e 1-e 0+e],[0 0 1 1-e 0+e 0+e],c2);patch([0 0 1 1-e 0+e 0+e],[0 1 1 1-e 1-e 0+e],c3);plot([0 1 1 0 0],[0 0 1 1 0]);
  Delays 1 : Subsystem
      mask Display: e = 0.06;c1 = [120 150 230]/255;c2 = ([120 150 230]+0)/383;c3 = ([120 150 230]+128)/383;patch([0 1 1 0],[0 0 1 1],c1);patch([0 1 1 1-e 1-e 0+e],[0 0 1 1-e 0+e 0+e],c2);patch([0 0 1 1-e 0+e 0+e],[0 1 1 1-e 1-e 0+e],c3);plot([0 1 1 0 0],[0 0 1 1 0]);disp('0');
  "LW{2,1}" : Subsystem
      mask Display: e = 0.06;c1 = [120 150 230]/255;c2 = ([120 150 230]+0)/383;c3 = ([120 150 230]+128)/383;patch([0 1 1 0],[0 0 1 1],c1);patch([0 1 1 1-e 1-e 0+e],[0 0 1 1-e 0+e 0+e],c2);patch([0 0 1 1-e 0+e 0+e],[0 1 1 1-e 1-e 0+e],c3);plot([0 1 1 0 0],[0 0 1 1 0]);disp('W');
  "b{2}" : Constant  Value=[1.563551636846649106615814162069000303745269775390625;-1.4978454032370667192708424408920109272003173828125;-1.3289200853858016415642850915901362895965576171875;-1.3380484106885879302950570490793325006961822509765625;1.2197333259574574260142298953724093735218048095703125;1.1147928880834481191186569049023091793060302734375;-0.97066732382520282129689803696237504482269287109375;0.7046617402704640209520903226803056895732879638671875;-0.6567680402391589122856885296641848981380462646484375;0.67998032338593217271949242785922251641750335693359375;-0.57488931654072772392538581698318012058734893798828125;0.435774831632942671877373186362092383205890655517578125;-0.252760446322219889392357572432956658303737640380859375;-0.165264473741079331858827572432346642017364501953125;0.1249133124195813404622157349876943044364452362060546875;0.235481255466414296506627579219639301300048828125;-0.34546312174978888176468672099872492253780364990234375;0.00553776421451674348561677874158704071305692195892333984375;-0.272752504203841839025557192144333384931087493896484375;-0.6898228184034904675314692212850786745548248291015625;-0.4228125065584309449917554957210086286067962646484375;-0.74044284692499606759241714826202951371669769287109375;-0.85896399666377842851971990967285819351673126220703125;0.84712433054146796251870910055004060268402099609375;-0.92684969300485076093565339760971255600452423095703125;1.0595597132729086542468621701118536293506622314453125;1.18603741583510302604054231778718531131744384765625;-1.3637969298273038276647639577277004718780517578125;-1.489532493625622233679450800991617143154144287109375;-1.5174593371481905901276832082658074796199798583984375]
      mask Display: e = 0.06;c1 = [120 150 230]/255;c2 = ([120 150 230]+0)/383;c3 = ([120 150 230]+128)/383;patch([0 1 1 0],[0 0 1 1],c1);patch([0 1 1 1-e 1-e 0+e],[0 0 1 1-e 0+e 0+e],c2);patch([0 0 1 1-e 0+e 0+e],[0 1 1 1-e 1-e 0+e],c3);plot([0 1 1 0 0],[0 0 1 1 0]);disp('b');
  netsum : Sum  Inputs=2  InputSameDT=on  SaturateOnIntegerOverflow=on  OutDataTypeStr=Inherit: Same as first input
      mask Display: e = 0.06;c1 = [120 150 230]/255;c2 = ([120 150 230]+0)/383;c3 = ([120 150 230]+128)/383;patch([0 1 1 0],[0 0 1 1],c1);patch([0 1 1 1-e 1-e 0+e],[0 0 1 1-e 0+e 0+e],c2);patch([0 0 1 1-e 0+e 0+e],[0 1 1 1-e 1-e 0+e],c3);plot([0 1 1 0 0],[0 0 1 1 0]);disp('+');
  tansig : neural/Transfer Functions/tansig
  "a{2}" : Outport  InitialOutput=[0;0;0;0;0;0;0;0;0;0;0;0;0;0;0;0;0;0;0;0;0;0;0;0;0;0;0;0;0;0]
      mask Display: e = 0.06;c1 = [120 230 180]/255;c2 = ([120 230 180]+0)/(256+128);c3 = ([120 230 180]+128)/(256+128);patch([0 1 1 0],[0 0 1 1],c1);patch([0 1 1 1-e 1-e 0+e],[0 0 1 1-e 0+e 0+e],c2);patch([0 0 1 1-e 0+e 0+e],[0 1 1 1-e 1-e 0+e],c3);plot([0 1 1 0 0],[0 0 1 1 0]);
  wires:
  "a{1} "/1 -> Delays 1/1("p{2}")
  Delays 1/1("pd{2,1}") -> "LW{2,1}"/1("ad{2,1}")
  "LW{2,1}"/1("lz{2,1}") -> netsum/1
  "b{2}"/1 -> netsum/2
  netsum/1 -> tansig/1
  tansig/1 -> "a{2}"/1

== system QuadrotorSimulink_no_memory/NN/Layer 3 ==
  "a{2} " : Inport  PortDimensions=30
      mask Display: e = 0.06;c1 = [120 230 180]/255;c2 = ([120 230 180]+0)/(256+128);c3 = ([120 230 180]+128)/(256+128);patch([0 1 1 0],[0 0 1 1],c1);patch([0 1 1 1-e 1-e 0+e],[0 0 1 1-e 0+e 0+e],c2);patch([0 0 1 1-e 0+e 0+e],[0 1 1 1-e 1-e 0+e],c3);plot([0 1 1 0 0],[0 0 1 1 0]);
  Delays 1 : Subsystem
      mask Display: e = 0.06;c1 = [120 150 230]/255;c2 = ([120 150 230]+0)/383;c3 = ([120 150 230]+128)/383;patch([0 1 1 0],[0 0 1 1],c1);patch([0 1 1 1-e 1-e 0+e],[0 0 1 1-e 0+e 0+e],c2);patch([0 0 1 1-e 0+e 0+e],[0 1 1 1-e 1-e 0+e],c3);plot([0 1 1 0 0],[0 0 1 1 0]);disp('0');
  "LW{3,2}" : Subsystem
      mask Display: e = 0.06;c1 = [120 150 230]/255;c2 = ([120 150 230]+0)/383;c3 = ([120 150 230]+128)/383;patch([0 1 1 0],[0 0 1 1],c1);patch([0 1 1 1-e 1-e 0+e],[0 0 1 1-e 0+e 0+e],c2);patch([0 0 1 1-e 0+e 0+e],[0 1 1 1-e 1-e 0+e],c3);plot([0 1 1 0 0],[0 0 1 1 0]);disp('W');
  "b{3}" : Constant  Value=[0.4971693472270863889406200541998259723186492919921875;0.944759804912518319497394259087741374969482421875]
      mask Display: e = 0.06;c1 = [120 150 230]/255;c2 = ([120 150 230]+0)/383;c3 = ([120 150 230]+128)/383;patch([0 1 1 0],[0 0 1 1],c1);patch([0 1 1 1-e 1-e 0+e],[0 0 1 1-e 0+e 0+e],c2);patch([0 0 1 1-e 0+e 0+e],[0 1 1 1-e 1-e 0+e],c3);plot([0 1 1 0 0],[0 0 1 1 0]);disp('b');
  netsum : Sum  Inputs=2  InputSameDT=on  SaturateOnIntegerOverflow=on  OutDataTypeStr=Inherit: Same as first input
      mask Display: e = 0.06;c1 = [120 150 230]/255;c2 = ([120 150 230]+0)/383;c3 = ([120 150 230]+128)/383;patch([0 1 1 0],[0 0 1 1],c1);patch([0 1 1 1-e 1-e 0+e],[0 0 1 1-e 0+e 0+e],c2);patch([0 0 1 1-e 0+e 0+e],[0 1 1 1-e 1-e 0+e],c3);plot([0 1 1 0 0],[0 0 1 1 0]);disp('+');
  purelin : neural/Transfer Functions/purelin
  "a{3}" : Outport  InitialOutput=[0;0]
      mask Display: e = 0.06;c1 = [120 230 180]/255;c2 = ([120 230 180]+0)/(256+128);c3 = ([120 230 180]+128)/(256+128);patch([0 1 1 0],[0 0 1 1],c1);patch([0 1 1 1-e 1-e 0+e],[0 0 1 1-e 0+e 0+e],c2);patch([0 0 1 1-e 0+e 0+e],[0 1 1 1-e 1-e 0+e],c3);plot([0 1 1 0 0],[0 0 1 1 0]);
  wires:
  "a{2} "/1 -> Delays 1/1("p{3}")
  Delays 1/1("pd{3,2}") -> "LW{3,2}"/1("ad{3,2}")
  "LW{3,2}"/1("lz{3,2}") -> netsum/1
  "b{3}"/1 -> netsum/2
  netsum/1 -> purelin/1
  purelin/1 -> "a{3}"/1

== system QuadrotorSimulink_no_memory/NN/Process Input 1 ==
  x : Inport  PortDimensions=5
      mask Display: e = 0.06;c1 = [120 230 180]/255;c2 = ([120 230 180]+0)/(256+128);c3 = ([120 230 180]+128)/(256+128);patch([0 1 1 0],[0 0 1 1],c1);patch([0 1 1 1-e 1-e 0+e],[0 0 1 1-e 0+e 0+e],c2);patch([0 0 1 1-e 0+e 0+e],[0 1 1 1-e 1-e 0+e],c3);plot([0 1 1 0 0],[0 0 1 1 0]);
  mapminmax : neural/Processing Functions/mapminmax  xmin=[0.206250000000000072164496600635;0.000591715976331361062992564292529;-1.24286750523964959456741513621e-05;0;-0.0107075553863898928486086958856]  xmax=[0.387500000000000011102230246252;0.0923076923076923128164139598084;5.35078896628240365906763187365e-05;0.453428937371301687964120219476;0.100496355467121947779851609539]  ymin=-1  ymax=1
  p : Outport  PortDimensions=5
      mask Display: e = 0.06;c1 = [120 230 180]/255;c2 = ([120 230 180]+0)/(256+128);c3 = ([120 230 180]+128)/(256+128);patch([0 1 1 0],[0 0 1 1],c1);patch([0 1 1 1-e 1-e 0+e],[0 0 1 1-e 0+e 0+e],c2);patch([0 0 1 1-e 0+e 0+e],[0 1 1 1-e 1-e 0+e],c3);plot([0 1 1 0 0],[0 0 1 1 0]);
  wires:
  x/1 -> mapminmax/1
  mapminmax/1 -> p/1

== system QuadrotorSimulink_no_memory/NN/Process Output 1 ==
  a : Inport  PortDimensions=2
      mask Display: e = 0.06;c1 = [120 230 180]/255;c2 = ([120 230 180]+0)/(256+128);c3 = ([120 230 180]+128)/(256+128);patch([0 1 1 0],[0 0 1 1],c1);patch([0 1 1 1-e 1-e 0+e],[0 0 1 1-e 0+e 0+e],c2);patch([0 0 1 1-e 0+e 0+e],[0 1 1 1-e 1-e 0+e],c3);plot([0 1 1 0 0],[0 0 1 1 0]);
  mapminmax_reverse : neural/Processing Functions/mapminmax_reverse  xmin=[-0.0387500000000000066613381477509;-0.00873707378433970748010661822036]  xmax=[0.0165451992159274009763780810545;0.00897959183673469572839476171566]  ymin=-1  ymax=1
  y : Outport  PortDimensions=2
      mask Display: e = 0.06;c1 = [120 230 180]/255;c2 = ([120 230 180]+0)/(256+128);c3 = ([120 230 180]+128)/(256+128);patch([0 1 1 0],[0 0 1 1],c1);patch([0 1 1 1-e 1-e 0+e],[0 0 1 1-e 0+e 0+e],c2);patch([0 0 1 1-e 0+e 0+e],[0 1 1 1-e 1-e 0+e],c3);plot([0 1 1 0 0],[0 0 1 1 0]);
  wires:
  a/1 -> mapminmax_reverse/1
  mapminmax_reverse/1 -> y/1

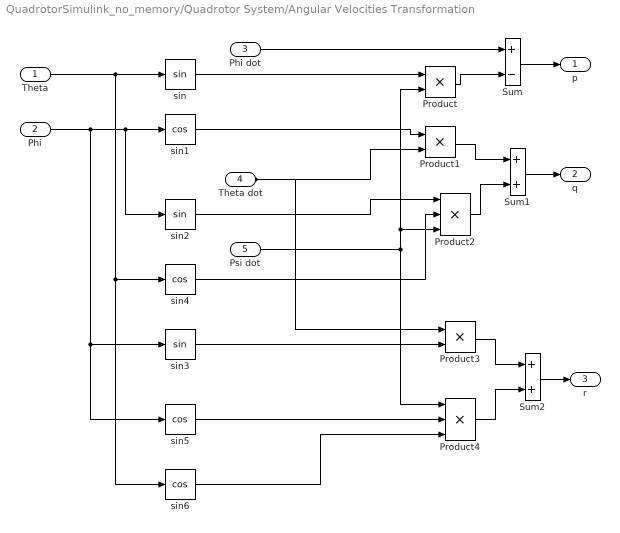
== system QuadrotorSimulink_no_memory/Quadrotor System/Angular Velocities Transformation ==
  Theta : Inport
  Phi : Inport  Port=2
  Phi dot : Inport  Port=3
  Theta dot : Inport  Port=4
  Psi dot : Inport  Port=5
  Product : Product  RndMeth=Zero
  Product1 : Product  RndMeth=Zero
  Product2 : Product  Inputs=3  RndMeth=Zero
  Product3 : Product  RndMeth=Zero
  Product4 : Product  Inputs=3  RndMeth=Zero
  Sum : Sum  Inputs=+-
  Sum1 : Sum
  Sum2 : Sum
  sin : Trigonometry
  sin{1,4..6} (4 alike) : Trigonometry  Operator=cos
  sin2 : Trigonometry
  sin3 : Trigonometry
  p : Outport  VectorParamsAs1DForOutWhenUnconnected=off
  q : Outport  Port=2  VectorParamsAs1DForOutWhenUnconnected=off
  r : Outport  Port=3  VectorParamsAs1DForOutWhenUnconnected=off
  wires:
  Phi dot/1 -> Sum/1
  Theta/1 -> sin4/1, sin6/1, sin/1
  sin/1 -> Product/1
  Psi dot/1 -> Product/2, Product2/3, Product4/1
  Product/1 -> Sum/2
  Sum/1 -> p/1
  Phi/1 -> sin1/1, sin2/1, sin3/1, sin5/1
  sin1/1 -> Product1/1
  Theta dot/1 -> Product1/2, Product3/1
  Product1/1 -> Sum1/1
  sin2/1 -> Product2/1
  sin4/1 -> Product2/2
  Product2/1 -> Sum1/2
  Sum1/1 -> q/1
  sin3/1 -> Product3/2
  sin5/1 -> Product4/2
  sin6/1 -> Product4/3
  Product3/1 -> Sum2/1
  Product4/1 -> Sum2/2
  Sum2/1 -> r/1

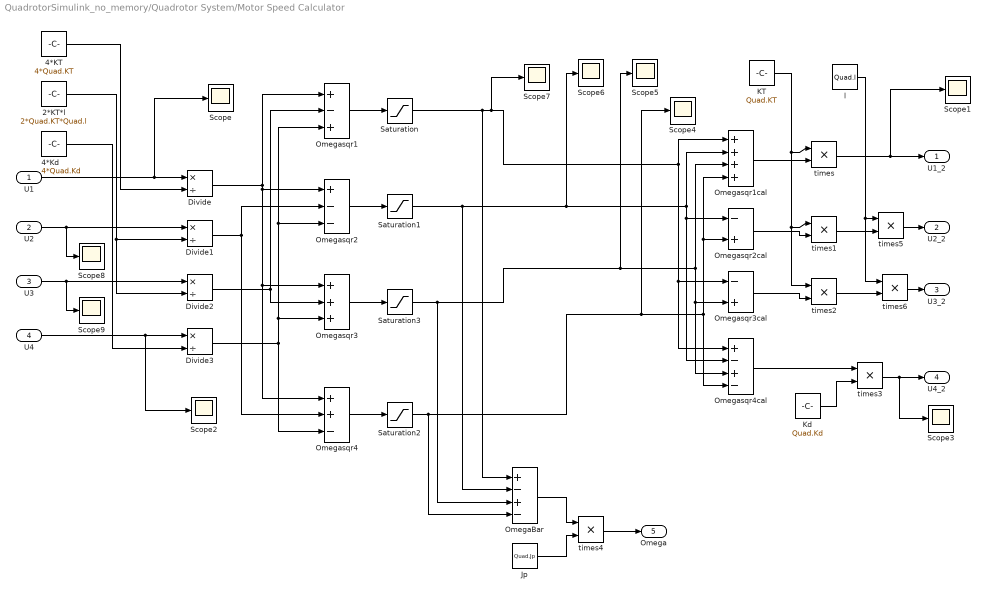
== system QuadrotorSimulink_no_memory/Quadrotor System/Motor Speed Calculator ==
  U1 : Inport
  U2 : Inport  Port=2
  U3 : Inport  Port=3
  U4 : Inport  Port=4
  2*KT*l : Constant  Value=2*Quad.KT*Quad.l
  4*KT : Constant  Value=4*Quad.KT
  4*Kd : Constant  Value=4*Quad.Kd
  Divide{,1..3} (4 alike) : Product  Inputs=*/
  Jp : Constant  Value=Quad.Jp
  KT : Constant  Value=Quad.KT
  Kd : Constant  Value=Quad.Kd
  OmegaBar : Sum  Inputs=+-+-
  Omegasqr1 : Sum  Inputs=+-+
  Omegasqr1cal : Sum  Inputs=++++
  Omegasqr2 : Sum  Inputs=+--
  Omegasqr2cal : Sum  Inputs=-+
  Omegasqr3 : Sum  Inputs=+++
  Omegasqr3cal : Sum  Inputs=-+
  Omegasqr4 : Sum  Inputs=++-
  Omegasqr4cal : Sum  Inputs=+-+-
  Saturation{,1..3} (4 alike) : Saturate  UpperLimit=Quad.max_motor_speed^2  LowerLimit=Quad.min_motor_speed^2  ZeroCross=off
  Scope{,1..9} (10 alike) : Scope
  l : Constant  Value=Quad.l
  times{,1..6} (7 alike) : Product  Inputs=**
  U1_2 : Outport  VectorParamsAs1DForOutWhenUnconnected=off
  U2_2 : Outport  Port=2  VectorParamsAs1DForOutWhenUnconnected=off
  U3_2 : Outport  Port=3  VectorParamsAs1DForOutWhenUnconnected=off
  U4_2 : Outport  Port=4  VectorParamsAs1DForOutWhenUnconnected=off
  Omega : Outport  Port=5  VectorParamsAs1DForOutWhenUnconnected=off
  wires:
  U1/1 -> Divide/1, Scope/1
  4*KT/1 -> Divide/2
  U2/1 -> Divide1/1, Scope8/1
  2*KT*l/1 -> Divide1/2, Divide2/2
  U3/1 -> Divide2/1, Scope9/1
  U4/1 -> Divide3/1, Scope2/1
  4*Kd/1 -> Divide3/2
  Divide/1 -> Omegasqr1/1, Omegasqr2/1, Omegasqr3/1, Omegasqr4/1
  Divide2/1 -> Omegasqr1/2, Omegasqr3/2
  Divide3/1 -> Omegasqr1/3, Omegasqr2/3, Omegasqr3/3, Omegasqr4/3
  Divide1/1 -> Omegasqr2/2, Omegasqr4/2
  OmegaBar/1 -> times4/1
  times4/1 -> Omega/1
  KT/1 -> times/1, times1/1, times2/1
  Omegasqr1cal/1 -> times/2
  Omegasqr2cal/1 -> times1/2
  Omegasqr3cal/1 -> times2/2
  Omegasqr4cal/1 -> times3/1
  Kd/1 -> times3/2
  times/1 -> U1_2/1, Scope1/1
  times3/1 -> U4_2/1, Scope3/1
  Jp/1 -> times4/2
  times5/1 -> U2_2/1
  times6/1 -> U3_2/1
  l/1 -> times5/1, times6/1
  times1/1 -> times5/2
  times2/1 -> times6/2
  Saturation/1 -> OmegaBar/1, Omegasqr1cal/1, Omegasqr3cal/1, Omegasqr4cal/1, Scope7/1
  Saturation2/1 -> OmegaBar/4, Omegasqr1cal/4, Omegasqr2cal/2, Omegasqr4cal/4, Scope4/1
  Saturation3/1 -> OmegaBar/3, Omegasqr1cal/3, Omegasqr3cal/2, Omegasqr4cal/3, Scope5/1
  Saturation1/1 -> OmegaBar/2, Omegasqr1cal/2, Omegasqr2cal/1, Omegasqr4cal/2, Scope6/1
  Omegasqr1/1 -> Saturation/1
  Omegasqr2/1 -> Saturation1/1
  Omegasqr3/1 -> Saturation3/1
  Omegasqr4/1 -> Saturation2/1

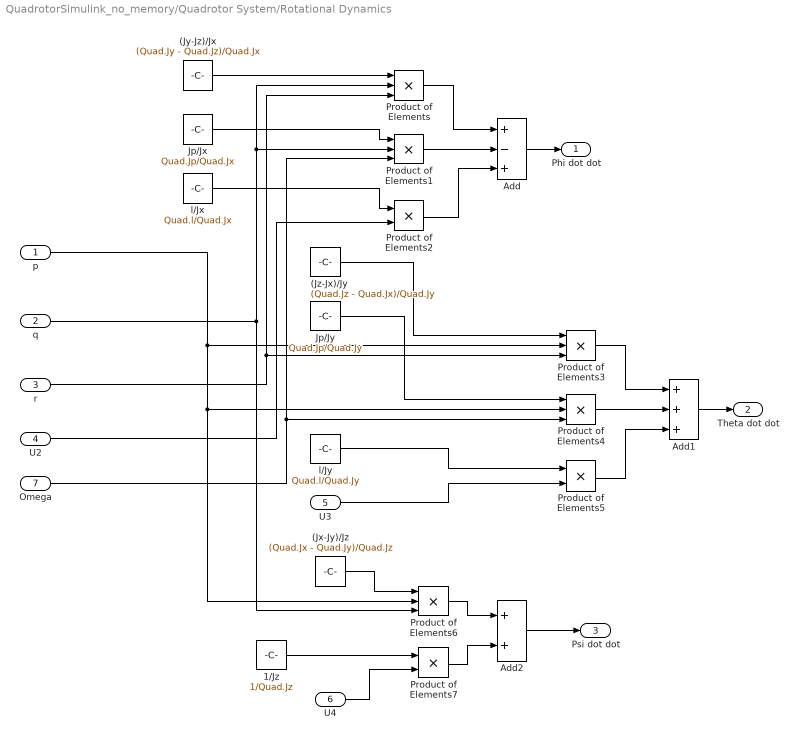
== system QuadrotorSimulink_no_memory/Quadrotor System/Rotational Dynamics ==
  p : Inport
  q : Inport  Port=2
  r : Inport  Port=3
  U2 : Inport  Port=4
  U3 : Inport  Port=5
  U4 : Inport  Port=6
  Omega : Inport  Port=7
  (Jx-Jy)/Jz : Constant  Value=(Quad.Jx - Quad.Jy)/Quad.Jz
  (Jy-Jz)/Jx : Constant  Value=(Quad.Jy - Quad.Jz)/Quad.Jx
  (Jz-Jx)/Jy : Constant  Value=(Quad.Jz - Quad.Jx)/Quad.Jy
  1/Jz : Constant  Value=1/Quad.Jz
  Add : Sum  Inputs=+-+
  Add1 : Sum  Inputs=+++
  Add2 : Sum
  Jp/Jx : Constant  Value=Quad.Jp/Quad.Jx
  Jp/Jy : Constant  Value=Quad.Jp/Quad.Jy
  Product of Elements{,1,3..4,6} (5 alike) : Product  Inputs=3
  Product of Elements2 : Product
  Product of Elements5 : Product
  Product of Elements7 : Product
  l/Jx : Constant  Value=Quad.l/Quad.Jx
  l/Jy : Constant  Value=Quad.l/Quad.Jy
  Phi dot dot : Outport  VectorParamsAs1DForOutWhenUnconnected=off
  Theta dot dot : Outport  Port=2  VectorParamsAs1DForOutWhenUnconnected=off
  Psi dot dot : Outport  Port=3  VectorParamsAs1DForOutWhenUnconnected=off
  wires:
  Product of Elements/1 -> Add/1
  Product of Elements1/1 -> Add/2
  Product of Elements2/1 -> Add/3
  Add/1 -> Phi dot dot/1
  (Jy-Jz)/Jx/1 -> Product of Elements/1
  q/1 -> Product of Elements/2, Product of Elements1/2, Product of Elements6/3
  r/1 -> Product of Elements/3, Product of Elements3/3
  Jp/Jx/1 -> Product of Elements1/1
  l/Jx/1 -> Product of Elements2/1
  U2/1 -> Product of Elements2/2
  Omega/1 -> Product of Elements1/3, Product of Elements4/3
  Product of Elements3/1 -> Add1/1
  Product of Elements4/1 -> Add1/2
  Product of Elements5/1 -> Add1/3
  Add1/1 -> Theta dot dot/1
  (Jz-Jx)/Jy/1 -> Product of Elements3/1
  Jp/Jy/1 -> Product of Elements4/1
  l/Jy/1 -> Product of Elements5/1
  U3/1 -> Product of Elements5/2
  p/1 -> Product of Elements3/2, Product of Elements4/2, Product of Elements6/2
  Product of Elements7/1 -> Add2/2
  Add2/1 -> Psi dot dot/1
  U4/1 -> Product of Elements7/2
  1/Jz/1 -> Product of Elements7/1
  (Jx-Jy)/Jz/1 -> Product of Elements6/1
  Product of Elements6/1 -> Add2/1
